simulink model "Short5thOrderInverseKin"  (R2023b)
settings: Solver=VariableStepAuto  StartTime=0.0  StopTime=300  RelTol=1e-3
libraries: dspnetwork x2
settings Model: Creator=skala  LastModifiedBy=jeric

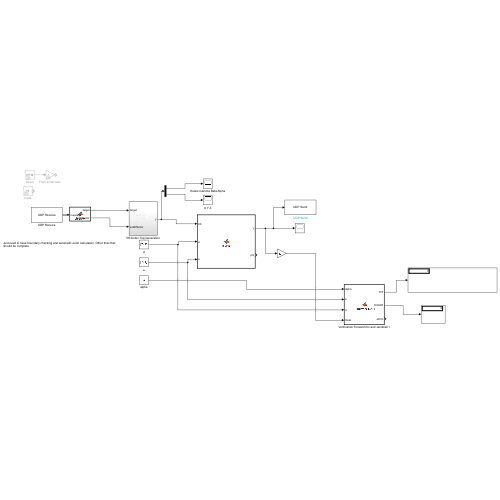
[thumbnail: Simulink's stored preview of the top-level diagram]
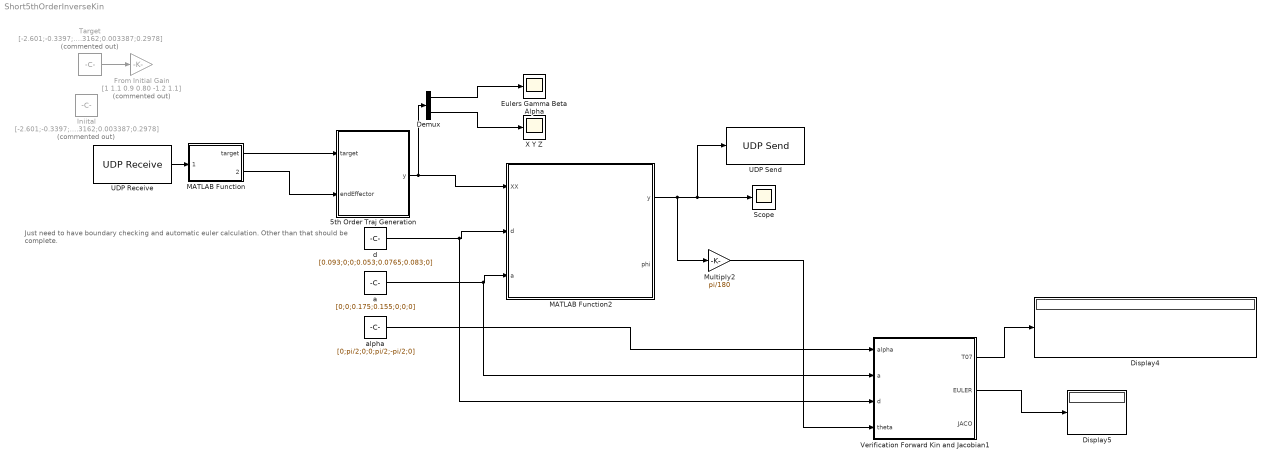
== system Short5thOrderInverseKin ==
  note: Just need to have boundary checking and automatic euler calculation. Other than that should be complete.
  5th Order Traj Generation : Subsystem
  Demux : Demux  Outputs=2
  Display4 : Display
  Display5 : Display
  Eulers Gamma Beta Alpha : Scope
  "From Initial Gain " : Gain  Commented=on  Gain=[1 1.1 0.9 0.80 -1.2 1.1]
  "Iniital " : Constant  Commented=on  Value=[-2.601;-0.3397;-1.7565;0.3162;0.003387;0.2978]
  MATLAB Function : MATLAB Function  TreatAsAtomicUnit=on
  MATLAB Function2 : MATLAB Function  TreatAsAtomicUnit=on
  Multiply2 : Gain  Gain=pi/180
  Scope : Scope
  Target : Constant  Commented=on  Value=[-2.601;-0.3397;-1.7565;0.3162;0.003387;0.2978]
  UDP Receive : dspnetwork/UDP Receive  localURL='0.0.0.0'  localPort=25566  remoteURL='0.0.0.0'  remotePort=-1  recvBufferSize=8192  dims=21  signalDatatype=double  isComplex=off  isVarSize=on  showBlockingTime=off  blockingTime=0  sampletime=.0001  blockPlatform=[]
      settings: LibrarySourceBlock=dspsrcs4/UDP Receive
  UDP Send : dspnetwork/UDP Send  remoteURL='127.0.0.1'  remotePort=25565  localURL='0.0.0.0'  localPortSource=Automatically determine  localPort=-1  sendBufferSize=8192  sampletime=-1  blockPlatform=[]  separateLengthPort=0
      settings: LibrarySourceBlock=dspsnks4/UDP Send
  Verification Forward Kin and Jacobian1 : MATLAB Function  TreatAsAtomicUnit=on
  X Y Z : Scope
  a : Constant  Value=[0;0;0.175;0.155;0;0;0]
  alpha : Constant  Value=[0;pi/2;0;0;pi/2;-pi/2;0]
  d : Constant  Value=[0.093;0;0;0.053;0.0765;0.083;0]
  wires:
  5th Order Traj Generation/1(y) -> Demux/1, MATLAB Function2/1(XX)
  d/1 -> Verification Forward Kin and Jacobian1/3(d), MATLAB Function2/2(d)
  a/1 -> Verification Forward Kin and Jacobian1/2(a), MATLAB Function2/3(a)
  MATLAB Function2/1(y) -> Multiply2/1, UDP Send/1, Scope/1
  alpha/1 -> Verification Forward Kin and Jacobian1/1(alpha)
  Multiply2/1 -> Verification Forward Kin and Jacobian1/4(theta)
  Verification Forward Kin and Jacobian1/1(T07) -> Display4/1
  Verification Forward Kin and Jacobian1/2(EULER) -> Display5/1
  Target/1 -> "From Initial Gain "/1
  Demux/1 -> Eulers Gamma Beta Alpha/1
  Demux/2 -> X Y Z/1
  UDP Receive/1 -> MATLAB Function/1(message)
  MATLAB Function/1(target) -> 5th Order Traj Generation/1(target)
  MATLAB Function/2(endEffector) -> 5th Order Traj Generation/2(endEffector)

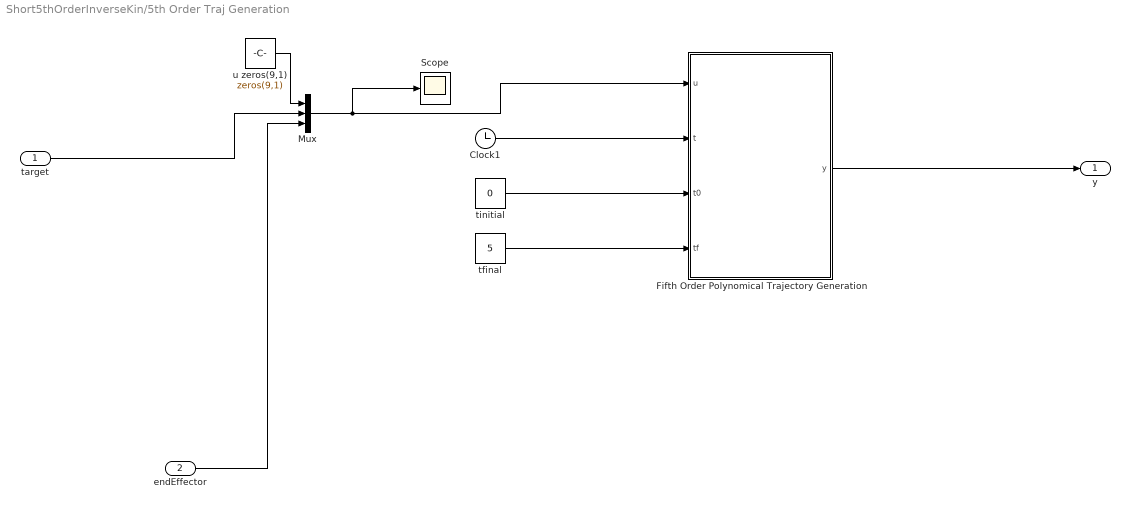
== system Short5thOrderInverseKin/5th Order Traj Generation ==
  target : Inport
  endEffector : Inport  Port=2
  Clock1 : Clock
  Fifth Order Polynomical Trajectory Generation : MATLAB Function  TreatAsAtomicUnit=on
  Mux : Mux  Inputs=3
  Scope : Scope
  tfinal : Constant  Value=5
  tinitial : Constant  Value=0
  u zeros(9,1) : Constant  Value=zeros(9,1)
  y : Outport
  wires:
  Mux/1 -> Scope/1, Fifth Order Polynomical Trajectory Generation/1(u)
  u zeros(9,1)/1 -> Mux/1
  tfinal/1 -> Fifth Order Polynomical Trajectory Generation/4(tf)
  Fifth Order Polynomical Trajectory Generation/1(y) -> y/1
  tinitial/1 -> Fifth Order Polynomical Trajectory Generation/3(t0)
  Clock1/1 -> Fifth Order Polynomical Trajectory Generation/2(t)
  target/1 -> Mux/2
  endEffector/1 -> Mux/3

== matlab function Short5thOrderInverseKin/MATLAB Function2 ==
  data: y output; XX input; d input; a input; phi output
function [y,phi]= invkin(XX, d,  a)
gamma=XX(1);beta=XX(2); alp=XX(3);
P=XX(4:6);
ROTg=[1 0 0; 0 cos(gamma) -sin(gamma); 0 sin(gamma) cos(gamma)];
ROTb=[cos(beta) 0 sin(beta); 0 1 0; -sin(beta) 0 cos(beta)];
ROTa=[cos(alp) -sin(alp) 0; sin(alp) cos(alp) 0; 0 0 1];
ROT=ROTa*ROTb*ROTg;
T07=[ROT P; 0 0 0 1];
d6=d(6); d4=d(4);
P6=T07(1:3,4);
k6=T07(1:3,3); m6=T07(1:3,1);
P5=P6-d6*k6;
x5=P5(1); y5=P5(2); 
%%mag5=sqrt(x5^2+y5^2);
%%theta1=asin(d4/mag5)+atan2(y5,x5);
%%% ALTERNATIVE
K1b=-y5; K2b=x5; K3b=d4;
Topb=sqrt((K2b^2+K1b^2-K3b^2));
theta1b=2*atan((K2b-Topb)/(K3b+K1b));
%%%
r0=[sin(theta1b);-cos(theta1b);0];
u56=cross(r0,k6); u56m=sqrt(u56(1)^2+u56(2)^2+u56(3)^2);
v56m=dot(r0,k6);
theta5=atan2(u56m,v56m);
%%%%
%%%theta2i=ini(2); theta3i=ini(3); theta4i=ini(4);
%%phi=theta2i+theta3i+theta4i-pi/2;
%%%% Calculation of phi
r1=[cos(theta1b);sin(theta1b);0];
k5=cross(r0,k6);
r11=cross(r1,k5); 
r12=dot(r1,k5);
mag11=sqrt(r11(1)^2+r11(2)^2+r11(3)^2);
phi=atan2(mag11,r12);
%phi=21*pi/180;
%%
a2=a(3); a3=a(4); d5=d(5); d1=d(1);
P5p=P5-d4*r0;
z5p=P5p(3); x5p=P5p(1); y5p=P5p(2);
xb=sqrt(x5p^2+y5p^2);
h=z5p-d1;
K1=2*a2*xb-2*a2*d5*cos(phi);
K2=2*a2*h-2*a2*d5*sin(phi);
K3=xb^2+h^2+a2^2+d5^2-a3^2-2*d5*h*sin(phi)-2*d5*xb*cos(phi);
Top=sqrt((K2^2+K1^2-K3^2));
theta2=2*atan((K2-Top)/(K3+K1));
%%%
K4=xb-a2*cos(theta2)-d5*cos(phi);
K5=a3*cos(theta2);
K6=a3*sin(theta2);
Top2=sqrt(K6^2+K5^2-K4^2);
theta3=2*atan((-K6+Top2)/(K4+K5));
theta4=phi-theta2-theta3+pi/2;
%%%
k5=[cos(phi)*cos(theta1b);cos(phi)*sin(theta1b);sin(phi)];
m5=cross(k6,k5);
%m6=T07(1:3,1);
xx=dot(m5,m6);
yyv=cross(m5,m6);
yy=sqrt(yyv(1)^2+yyv(2)^2+yyv(3)^2);
theta6a=atan2(yy,xx);
%theta6b=acos(xx);
%theta6=asin(yy);

y = [theta1b;theta2;theta3;theta4;theta5;theta6a]*180/pi;

== matlab function Short5thOrderInverseKin/MATLAB Function ==
  data: message input; target output; endEffector output
function [target, endEffector] = Unpack(message)

target = [message(13:15); message(10:12)];
endEffector = [message(19:21); message(16:18)];

== matlab function Short5thOrderInverseKin/Verification Forward Kin and Jacobian1 ==
  data: alpha input; T07 output; EULER output; a input; d input; theta input; JACO output
function [T07,EULER,JACO]= FORWANDJAC(alpha,a,d,theta)
%format long
%theta1=theta(1); theta2=theta(2); theta3=theta(3); 
%theta4=theta(4); theta5= theta(5); theta6=theta(6); 
P=[0;0;1];
%
T01=DHPM(alpha(1),a(1),d(1),theta(1));
e1=T01(1:3,1:3)*P;
%
T12=DHPM(alpha(2),a(2),d(2), theta(2));
T02=T01*T12;
e2=T02(1:3,1:3)*P;
%
T23=DHPM(alpha(3), a(3),d(3), theta(3));
T03=T02*T23;
e3=T03(1:3,1:3)*P;
%
T34=DHPM(alpha(4), a(4),d(4), theta(4));
T04=T03*T34;
e4=T04(1:3,1:3)*P;
%
T45=DHPM(alpha(5), a(5),d(5), theta(5));
T05=T04*T45;
e5=T05(1:3,1:3)*P;
%
T56=DHPM(alpha(6),a(6),d(6), theta(6)) ;
T06=T05*T56;
e6=T06(1:3,1:3)*P;
%
T67=DHPM(alpha(7), a(7),d(7),0);
T07=T06*T67;
P67L=T67(1:3,4);
P67=T07(1:3,1:3)*P67L;
%
T57=T56*T67;
P57L=T57(1:3,4);
P57=T05(1:3,1:3)*P57L;
%
T47=T45*T57;
P47L=T47(1:3,4);
P47=T04(1:3,1:3)*P47L;
%
T37=T34*T47;
P37L=T37(1:3,4);
P37=T03(1:3,1:3)*P37L;
%
T27=T23*T37;
P27L=T27(1:3,4);
P27=T02(1:3,1:3)*P27L;
%
T17=T12*T27;
P17L=T17(1:3,4);
P17=T01(1:3,1:3)*P17L;
%
T07=T01*T17;
P07=T07(1:3,4);
  beta=atan2(-T07(3,1),sqrt(T07(1,1)^2+T07(2,1)^2));
  if beta==pi/2
     alph=0.0;
     gamma=atan2(T07(1,2),T07(2,2));
  elseif beta==-pi/2
      alph=0.0;
      gamma=-atan2(T07(1,2),T07(2,2));
  else
  cb=cos(beta);
  alph=atan2(T07(2,1)/cb, T07(1,1)/cb);
  gamma=atan2(T07(3,2)/cb, T07(3,3)/cb);
  end
  EULER=[gamma;beta;alph]*180/pi;

JACT=[e1,e2,e3,e4,e5,e6];
b1=cross(e1,P17);
b2=cross(e2,P27);
b3=cross(e3,P37);
b4=cross(e4,P47);
b5=cross(e5,P57);
b6=cross(e6,P67);
JACB=[b1,b2,b3,b4,b5,b6];
JACO=[JACT;JACB];



function T=DHPM(alpha, a, d, theta)

T_xAlpha=[1 0 0 0 ;0 cos(alpha) -sin(alpha) 0 ;0 sin(alpha) cos(alpha) 0;0 0 0 1];
T_xA=[1 0 0 a;0 1 0 0;0 0 1 0;0 0 0 1];
T_zD=[1 0 0 0;0 1 0 0;0 0 1 d;0 0 0 1];
T_zTheta=[cos(theta) -sin(theta) 0 0;sin(theta) cos(theta) 0 0;0 0 1 0;0 0 0 1];
T=T_xAlpha*T_xA*T_zD*T_zTheta;

== matlab function Short5thOrderInverseKin/5th Order Traj Generation/Fifth Order Polynomical Trajectory Generation ==
  data: u input; y output; t input; t0 input; tf input
function y = TrajectoryGeneration(u, t, t0, tf)
%tf = 5;
%t0 = 0;
endEffector = u(16:21);
target = u(10:15);
A = [t0^5, t0^4, t0^3, t0^2, t0, 1;
5*t0^4, 4*t0^3, 3*t0^2, 2*t0, 1, 0;
20*t0^3, 12*t0^2, 6*t0, 2, 0, 0;
tf^5, tf^4, tf^3, tf^2, tf, 1;
5*tf^4, 4*tf^3, 3*tf^2, 2*tf, 1, 0;
20*tf^3, 12*tf^2, 6*tf, 2, 0, 0;];
row1 = endEffector(1:6)';
row2 = target(1:6)';
B = [row1;
0 0 0 0 0 0;
0 0 0 0 0 0;
row2;
0 0 0 0 0 0;
0 0 0 0 0 0;];
C = A \ B;
r = [t^5, t^4, t^3, t^2, t, 1];
rotation = [dot(r, C(1:6, 1));
dot(r, C(1:6, 2));
dot(r, C(1:6, 3));];
position = [dot(r, C(1:6, 4));
dot(r, C(1:6, 5));
dot(r, C(1:6, 6));];
y = [rotation; position];
%y = u;
